simulink model "RetailerInventory"  (R2017b)
settings: Solver=ode4  StartTime=0.0  StopTime=60  FixedStep=0.1  RelTol=1e-3
settings Model: Creator="ASUS  N551JW"  LastModifiedBy="ASUS  N551JW"

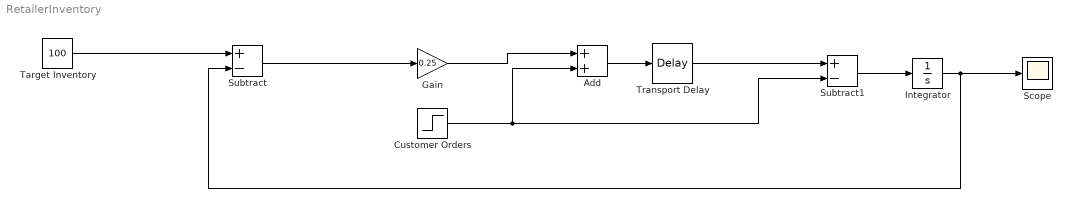
== system RetailerInventory ==
  Add : Sum
  "Customer Orders " : Step  Time=30  Before=60  After=80  SampleTime=0
  Gain : Gain  Gain=0.25
  Integrator : Integrator  InitialCondition=40
  Scope : Scope
  Subtract : Sum  Inputs=+-
  Subtract1 : Sum  Inputs=+-
  "Target Inventory " : Constant  Value=100
  Transport Delay : TransportDelay  DelayTime=4
  wires:
  "Target Inventory "/1 -> Subtract/1
  Subtract/1 -> Gain/1
  Gain/1 -> Add/1
  "Customer Orders "/1 -> Subtract1/2, Add/2
  Add/1 -> Transport Delay/1
  Transport Delay/1 -> Subtract1/1
  Subtract1/1 -> Integrator/1
  Integrator/1 -> Scope/1, Subtract/2
